simulink subsystem "EnergyElectroThermal"  (R2024b)
settings: Solver=VariableStepAuto  StartTime=0.0  StopTime=10.0  RelTol=1e-3
settings Model: Creator=jjha  LastModifiedBy=jjha
settings RTWCC: GPUComputeCapability=3.5

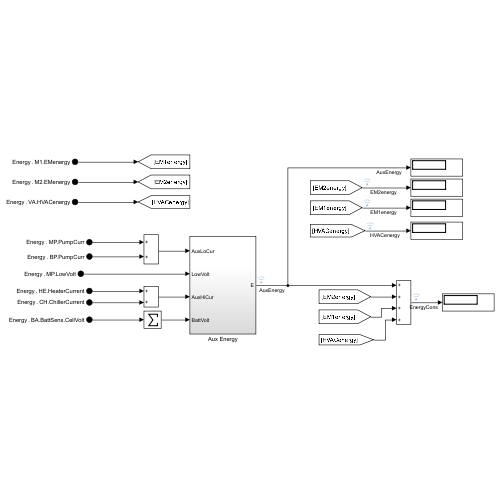
[thumbnail: Simulink's stored preview of the top-level diagram]
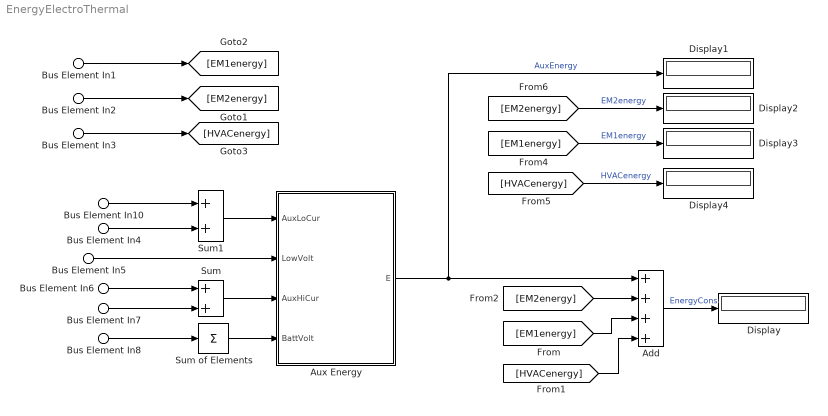
== system EnergyElectroThermal ==
  Bus Element In1 : Inport  PortName=Energy  Element=M1.EMenergy
  Bus Element In2 : Inport  PortName=Energy  Element=M2.EMenergy
  Bus Element In3 : Inport  PortName=Energy  Element=VA.HVACenergy
  Bus Element In10 : Inport  PortName=Energy  Element=MP.PumpCurr
  Bus Element In5 : Inport  PortName=Energy  Element=MP.LowVolt
  Bus Element In6 : Inport  PortName=Energy  Element=HE.HeaterCurrent
  Bus Element In7 : Inport  PortName=Energy  Element=CH.ChillerCurrent
  Bus Element In8 : Inport  PortName=Energy  Element=BA.BattSens.Cellvolt
  Bus Element In4 : Inport  PortName=Energy  Element=BP.PumpCurr
  Add : Sum  Inputs=++++
  Aux Energy : Subsystem
  Display{,1..4} (5 alike) : Display
  Sum : Sum
  Sum of Elements : Sum  Inputs=+
  Sum1 : Sum
  wires:
  [EM2energy] -> Add/2
  [EM1energy] -> Add/3
  [HVACenergy] -> Add/4
  Add/1 -> Display/1  "EnergyCons"
  Aux Energy/1(E) -> Add/1, Display1/1  "AuxEnergy"
  [EM2energy] -> Display2/1  "EM2energy"
  [EM1energy] -> Display3/1  "EM1energy"
  [HVACenergy] -> Display4/1  "HVACenergy"
  Bus Element In3/1 -> [HVACenergy]
  Bus Element In7/1 -> Sum/2
  Bus Element In5/1 -> Aux Energy/2(LowVolt)
  Sum1/1 -> Aux Energy/1(AuxLoCur)
  Sum/1 -> Aux Energy/3(AuxHiCur)
  Bus Element In6/1 -> Sum/1
  Bus Element In10/1 -> Sum1/1
  Bus Element In4/1 -> Sum1/2
  Bus Element In8/1 -> Sum of Elements/1
  Sum of Elements/1 -> Aux Energy/4(BattVolt)
  Bus Element In2/1 -> [EM2energy]
  Bus Element In1/1 -> [EM1energy]

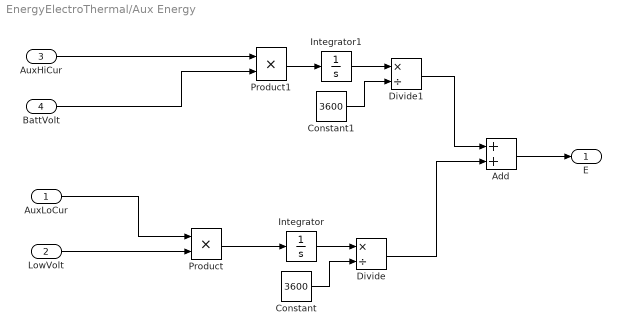
== system EnergyElectroThermal/Aux Energy ==
  AuxLoCur : Inport
  LowVolt : Inport  Port=2
  AuxHiCur : Inport  Port=3
  BattVolt : Inport  Port=4
  Add : Sum
  Constant : Constant  Value=3600
  Constant1 : Constant  Value=3600
  Divide : Product  Inputs=*/
  Divide1 : Product  Inputs=*/
  Integrator : Integrator  ZeroCross=off
  Integrator1 : Integrator  ZeroCross=off
  Product : Product
  Product1 : Product
  E : Outport
  wires:
  BattVolt/1 -> Product1/2
  Divide/1 -> Add/2
  Divide1/1 -> Add/1
  Product1/1 -> Integrator1/1
  Constant1/1 -> Divide1/2
  Integrator1/1 -> Divide1/1
  AuxHiCur/1 -> Product1/1
  Product/1 -> Integrator/1
  Integrator/1 -> Divide/1
  Constant/1 -> Divide/2
  LowVolt/1 -> Product/2
  Add/1 -> E/1
  AuxLoCur/1 -> Product/1
